simulink model "part4c"  (R2018a)
settings: Solver=VariableStepAuto  StartTime=0.0  StopTime=5000  RelTol=1e-3
values from neighbouring files (symbols this model uses):
  c = 16    [variables.m]
  kout = 0.1587    [variables.m]
  qin = 10*.134/60    (= 0.0223333333333)    [variables.m]
settings Model: Creator=jschm  LastModifiedBy=jschm

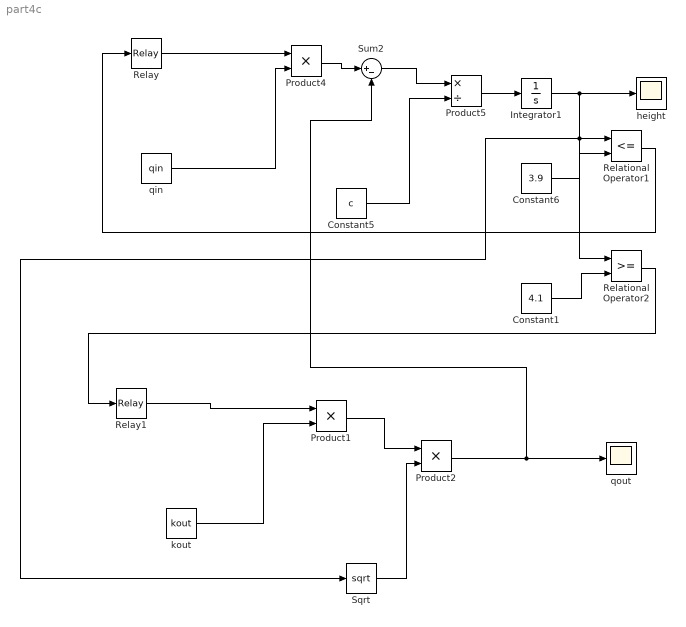
== system part4c ==
  Constant1 : Constant  Value=4.1
  Constant5 : Constant  Value=c
  Constant6 : Constant  Value=3.9
  Integrator1 : Integrator  InitialCondition=4
  Product1 : Product
  Product2 : Product
  Product4 : Product
  Product5 : Product  Inputs=*/
  Relational Operator1 : RelationalOperator  Operator=<=  OutDataTypeStr=boolean  RndMeth=Simplest
  Relational Operator2 : RelationalOperator  OutDataTypeStr=boolean  RndMeth=Simplest
  Relay : Relay
  Relay1 : Relay
  Sqrt : Sqrt  SaturateOnIntegerOverflow=on
  Sum2 : Sum  Inputs=|+-
  height : Scope
  "kout " : Constant  Value=kout
  "qin " : Constant  Value=qin
  qout : Scope
  wires:
  Relay1/1 -> Product1/1
  "kout "/1 -> Product1/2
  Product1/1 -> Product2/1
  Product2/1 -> Sum2/2, qout/1
  Integrator1/1 -> height/1, Relational Operator1/1, Relational Operator2/1, Sqrt/1
  Sqrt/1 -> Product2/2
  Constant5/1 -> Product5/2
  Relay/1 -> Product4/1
  Product4/1 -> Sum2/1
  Product5/1 -> Integrator1/1
  Constant6/1 -> Relational Operator1/2
  "qin "/1 -> Product4/2
  Sum2/1 -> Product5/1
  Relational Operator1/1 -> Relay/1
  Constant1/1 -> Relational Operator2/2
  Relational Operator2/1 -> Relay1/1
